simulink model "ee_igbt_thermal"  (R2021a)
settings: Solver=VariableStepAuto  StartTime=0.0  StopTime=t_sim  RelTol=1e-3  EnableMultiTasking=on
PreLoadFcn:
  | Vge = 10;
  | Vce_min = 0;
  | Vce_max = 5;
  | t_sim = 1;
  | T = 25;
StopFcn:
  | ee_addSimlogTimeStamp(bdroot)
libraries: fl_lib x4, nesl_utility x3, ee_lib x1, simulink x1
CloseFcn:
  | try,close(h1_ee_igbt_thermal),end
  | clear h1_ee_igbt_thermal
  | try,close(h2_ee_igbt_thermal),end
  | clear h2_ee_igbt_thermal
  | 
  | clear simlog_ee_igbt_thermal
  | clear logsout_ee_igbt_thermal
  | clear Ic IcVce10V IcVce12V IcVce15V IcVce20V IcVce8V Ic_mat Ic_max ModelName T Vce Vce_max Vce_min Vce_vec Vge Vge_vec i legend_info plot_colors t_sim tout
Description:
  | IGBT Thermal Characteristics
settings Model: FPTRunName=Active  ExtModeAutoUpdateStatusClock=off  Creator=The MathWorks, Inc.  LastModifiedBy=The MathWorks, Inc.
settings SolverCC: AlgebraicLoopSolver=TrustRegion
settings DataIOCC: LimitDataPoints=on  MaxDataPoints=10000  SaveFormat=Array  ReturnWorkspaceOutputs=off  SignalLoggingName=logsout_ee_igbt_thermal  OutputOption=SpecifiedOutputTimes  OutputTimes=[0:t_sim/100:t_sim]  Refine=5
settings OptimizationCC: ExpressionDepthLimit=2147483647  InitFltsAndDblsToZero=on  LifeSpan=inf
settings DebuggingCC: SaveWithParameterizedLinksMsg=none  UnderspecifiedInitializationDetection=Classic  MergeDetectMultiDrivingBlocksExec=none  SignalResolutionControl=TryResolveAllWithWarning  FcnCallInpInsideContextMsg=warning  StateNameClashWarn=warning  SFUnexpectedBacktrackingDiag=warning  SFNoUnconditionalDefaultTransitionDiag=warning  SFExecutionAtInitializationDiag=none  SFMachineParentedDataDiag=warning  ArithmeticOperatorsInVariantConditions=warning
settings HardwareCC: ProdBitPerPointer=32  ProdBitPerSizeT=32  ProdBitPerPtrDiffT=32  ProdLargestAtomicFloat=None  ProdIntDivRoundTo=Undefined  ProdEndianess=Unspecified  ProdWordSize=32  ProdHWDeviceType=32-bit Generic
settings ModelReferenceCC: PropagateSignalLabelsOutOfModel=off
settings SFSimCC: SimUseLocalCustomCode=off  CustomCodeUndefinedFunction=UseInterfaceOnly
settings RTWCC: RTWUseLocalCustomCode=off
settings CodeAppCC: StateflowObjectComments=on
settings GRTTargetCC: TargetFcnLib=ansi_tfl_tmw.mat  TargetLangStandard=C89/C90 (ANSI)  CombineOutputUpdateFcns=off  GRTInterface=on
settings ConfigComp: CovMetricSettings=dw  CovSaveCumulativeToWorkspaceVar=on  CovSaveSingleToWorkspaceVar=on  CovExternalEMLEnable=off  CovSFcnEnable=off
settings SimscapeCC: SimscapeLogType=all  SimscapeLogSimulationStatistics=on  SimscapeLogName=simlog_ee_igbt_thermal  SimscapeLogDataHistory=10000

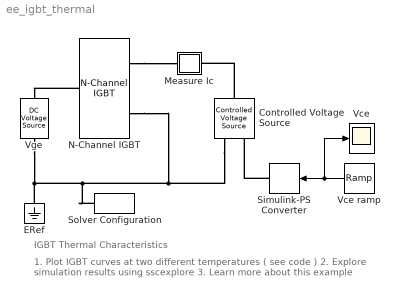
== system ee_igbt_thermal ==
  note: IGBT Thermal Characteristics
  note: 1. Plot IGBT curves at two different temperatures ( see code )
      | 2. Explore simulation results using sscexplore
      | 3. Learn more about this example
  Controlled Voltage Source : fl_lib/Electrical/Electrical Sources/Controlled Voltage Source
  ERef : fl_lib/Electrical/Electrical Elements/Electrical Reference
  Measure Ic : Subsystem
      mask Display: disp('i')
  N-Channel IGBT : ee_lib/Semiconductors & Converters/N-Channel IGBT  model_type=1  Ices=2 mA  Vces=600 V  Vth=7.1 V  Vce_sat=2.7 V  Ice_sat=400 A  Vge_sat=10 V  ec=2.5  Tmeas=25 degC  Vge_vec=[ -2 6 7 8 10 12 15 20 ] V  Vce_vec=[ -1 0 0.5 1 1.5 2 2.5 3 3.5 4 ] V  T_vec=[25, 125] degC  Ic_mat=[ -1.015e-5 1.35e-8 4.7135e-4 5.092e-4 5.105e-4 5.117500000000001e-4 5.1299e-4 5.1423e-4 5.1548e-4 5.1672e-4; -9.986899999999999e-6 1.35e-8 4.7135e-4 5.092e-4 5.105e-4 5.117500000000001e-4 5.1299e-4 5.1423e-4 5.1548e-4 5.1672e-4; -9.955e-6 1.35e-8 0.0065225 3.3324 48.154 93.661 105.52 105.72 105.93 106.14; -9.955e-6 1.35e-8 0.0065235 3.5783 70.264 166.33 252.4 317.67 353.38 357.39; -9.955e-6 1.35e-8 0.006524 3.7206 89.17100000000001 228.09 371.63 511.02 642.6900000000001 764.04; -9.9549e-6 1.35e-8 0.0065242 3.7716 97.79300000000001 256.21 424.27 592.92 759.2 921.52; -9.9549e-6 1.35e-8 0.0065243 3.8067 104.52 278.11 464.6 654.37 844.5700000000001 1.0339e+3; -9.9549e-6 1.35e-8 0.0065244 3.8324 109.92 295.67 496.54 702.28 909.96 1.1183e+3 ] A  Ic_mat_3D=zeros(8, 10, 2) A  C_param=1  C_GE=23.7 nF  C_GC=2.7 nF  C_CE=0 nF  C_ies=26.4 nF  C_res=2.7 nF  C_oes=0 nF  C_GE_vec=[ 25 31 26.5 24.9 25 24.9 24.6 24.7 24.8 ] nF  C_GC_vec=[ 55 9 5.5 3.1 2.5 2.1 1.9 1.8 1.7 ] nF  C_CE_vec=[ 5 11 6.5 4.9 3.5 2.7 2.1 1.7 1.4 ] nF  C_ies_vec=[ 80 40 32 28 27.5 27 26.5 26.5 26.5 ] nF  C_res_vec=[ 55 9 5.5 3.1 2.5 2.1 1.9 1.8 1.7 ] nF  C_oes_vec=[ 55 20 12 8 6 4.8 4 3.5 3.1 ] nF  C_Vce_vec=[ 0 1 2 5 10 15 20 25 30 ] V  charge_linearity_param=1  C_OX=20 nF  V_C_OX=-5 V  TF=0 us  VAF=60 V  RC=0.0001 Ohm  RE=0.0017 Ohm  RG=0.001 Ohm  BF=50  T_param=2  Ices_T2=50 mA  EG=1.11 eV  Vce_sat_T2=3 V  Tmeas2=125 degC  XTI=3  BEX=-2.5  RG_alpha=0 1/K  Tdevice=T degC  Tdevice_3D=25 degC  thermal_network_parameterization=ee.enum.thermalNetworkTopology.cauer  Rth=[0, 10] K/W  Rth_Foster=[4, 6] K/W  thermal_mass_parameterization=ee.enum.thermalNetwork.timeconstant  thermal_mass=[0, 1] J/K  thermal_mass_Foster=[1.5, 3] J/K  thermal_time_constant=[0, 10] s  thermal_time_constant_Foster=[6, 18] s  thermal_mass_initial_temperatures=[25, 25] degC  Ic_vec1=[0, 10, 50, 100, 200, 400, 600] A  Vce_vec1=[0, 1.1, 1.3, 1.45, 1.75, 2.25, 2.7] V  Rmiller=0.1 Ohm  Goff=1e-5 1/Ohm  t_on=0.07 us  t_rise=0.7 us  t_off=0.2 us  t_fall=0.5 us  v_meas=300 V  vStartTurnOn_specify=off  vStartTurnOn_priority=None  vStartTurnOn=1 V  tStartTurnOn_specify=off  tStartTurnOn_priority=None  tStartTurnOn=0 s  vStartTurnOff_specify=off  vStartTurnOff_priority=None  vStartTurnOff=0.5 V  tStartTurnOff_specify=off  tStartTurnOff_priority=None  tStartTurnOff=0 s  Tj_vec1=[298.15, 398.15] K  Vce_mat1=[0, 1.1, 1.3, 1.45, 1.75, 2.25, 2.7; 0, 1, 1.15, 1.35, 1.7, 2.35, 3] V  E_turn_on_mat1=[0, .2, 1, 2, 4, 8, 15; 0, .3, 1.3, 2.5, 5, 11, 18] * 1e-3 J  E_turn_off_mat1=[0, .3, 1.5, 3, 6, 15, 25; 0, .7, 3.3, 6.5, 13, 25, 35] * 1e-3 J  iStartTurnOff_specify=off  iStartTurnOff_priority=None  iStartTurnOff=0 A  Tdevice_specify=off  Tdevice_priority=None
      settings: SourceProductBaseCode=PS  InternalSimscapePortConfiguration="{\"Bottom\":[],\"Left\":[{\"id\":\"G\",\"label\":\"\",\"type\":\"foundation.electrical.electrical\"}],\"Right\":[{\"id\":\"C\",\"label\":\"\",\"type\":\"foundation.electrical.electrical\"},{\"id\":\"E\",\"label\":\"\",\"type\":\"foundation.electrical.electrical\"}],\"Top\":[]}"
  Simulink-PS Converter : nesl_utility/Simulink-PS Converter  PhysicalDomain=network_engine_domain  SubClassName=ps_input  LeftPortType=input  RightPortType=output  PseudoPeriodic=off  Frequencies=[]  NoiseDistribution=none  NoiseParameters=[]  Unit=1  AffineConversion=off  FilteringAndDerivatives=zero  SimscapeFilterOrder=1  InputFilterTimeConstant=.001  UdotUserProvided=0
      settings: SourceProductBaseCode=PW,SS
  Solver Configuration : nesl_utility/Solver Configuration  PhysicalDomain=network_engine_domain  SubClassName=solver  LeftPortType=input  RightPortType=generic  Tones=[]  Harmonics=[]  SimulateNoise=off  Profile=off  UseLocalSampling=off  EnableSwitchedLinearOptims=on  FrequencyDomain=off  UseCCode=off  RelTol=0.001  AbsTol=1e-06  MinStep=1e-09  ToWorkspace=off  RevertToSquareIcSolve=off  NumHomotopyIterations=100  PhasorMode=off  PhasorModeNumHarmonics=1  DoDC=on  ResidualTolerance=1e-9  UseLocalSolver=off  LocalSolverChoice=NE_BACKWARD_EULER_ADVANCER  LocalSolverSampleTime=.001  DoFixedCost=off  MaxNonlinIter=3  MaxModeIter=2  ComputeImpulses=off  ImpulseIterations=2  LinearAlgebra=auto  EquationFormulation=NE_TIME_EF  DelaysMemoryBudget=1024  AutomaticFiltering=on  FilteringTimeConstant=0.001  PartitionStorageMethod=AS_NEEDED  PartitionMemoryBudget=1024  PartitionMethod=FAST
      settings: SourceProductBaseCode=PW,SS
  Vce : Scope
  Vce ramp : simulink/Sources/Ramp  slope=(Vce_max-Vce_min)/t_sim  start=0  InitialOutput=Vce_min
  Vge : fl_lib/Electrical/Electrical Sources/DC Voltage Source  v0=Vge V
  wires:
  Vce ramp/1 -> Vce/1, Simulink-PS Converter/1
  connections:
  Controlled Voltage Source/LConn1 -- Measure Ic/RConn1
  Simulink-PS Converter/RConn1 -- Controlled Voltage Source/RConn1
  Controlled Voltage Source/RConn2 -- N-Channel IGBT/RConn2 -- Solver Configuration/RConn1 -- Vge/RConn1 -- ERef/LConn1
  N-Channel IGBT/RConn1 -- Measure Ic/LConn1
  N-Channel IGBT/LConn1 -- Vge/LConn1

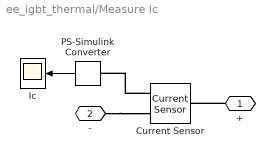
== system ee_igbt_thermal/Measure Ic ==
  Current Sensor : fl_lib/Electrical/Electrical Sensors/Current Sensor
  Ic : Scope
  PS-Simulink Converter : nesl_utility/PS-Simulink Converter  PhysicalDomain=network_engine_domain  SubClassName=ps_output  LeftPortType=input  RightPortType=output  PseudoPeriodic=off  Frequencies=[]  Unit=1  AffineConversion=off
      settings: SourceProductBaseCode=PW,SS
  + : PMIOPort  Side=Right
  - : PMIOPort  Port=2  Side=Left
  wires:
  PS-Simulink Converter/1 -> Ic/1
  connections:
  +/RConn1 -- Current Sensor/LConn1
  -/RConn1 -- Current Sensor/RConn2
  Current Sensor/RConn1 -- PS-Simulink Converter/LConn1
